simulink model "simulink_4"  (R2025b)
settings: Solver=ode45  StartTime=0.0  StopTime=0.5  MaxStep=1e-4  RelTol=1e-3
values from neighbouring files (symbols this model uses):
  A = [ -k1/(2*sqrt(x1e)),      0 ... (first row only)    [main.m]
  alpha = alpha_tau / tau    [main.m]
  B = [ k4; 0 ]    [main.m]
  C = [ 0, 1 ]    [main.m]
  D = 0    [main.m]
  Kr = 60    [main.m]
  tau = (M_star - cos(phi_rad)) / (wc_des * sin(phi_rad))    [main.m]
settings Model: Creator=porpo  LastModifiedBy=porpo

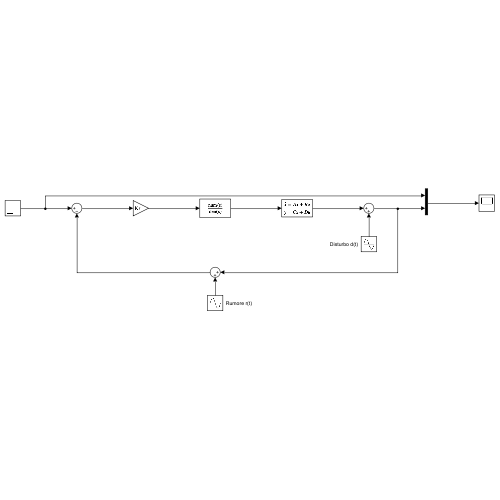
[thumbnail: Simulink's stored preview of the top-level diagram]
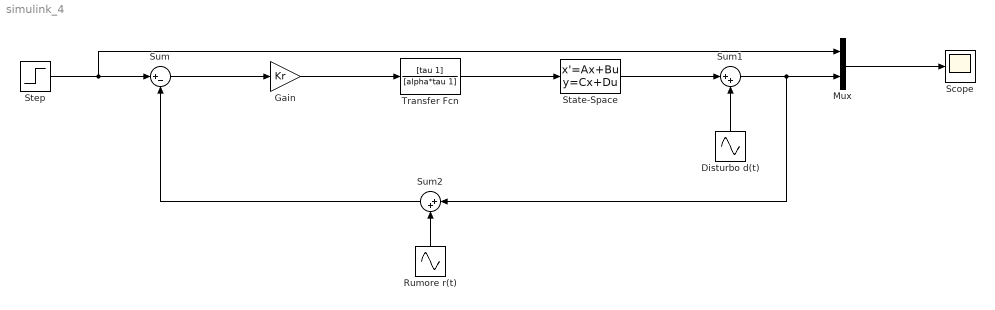
== system simulink_4 ==
  Disturbo d(t) : Sin  Amplitude=0  SampleTime=0
  Gain : Gain  Gain=Kr
  Mux : Mux  Inputs=2
  Rumore r(t) : Sin  Amplitude=0  SampleTime=0
  Scope : Scope
      settings: ActiveDisplayYMinimum=-0.95624767179996484  ActiveDisplayYMaximum=4.7591730752840817
  State-Space : StateSpace  A=A  B=B  C=C  D=D  InitialCondition=0
  Step : Step  Time=0  After=3  SampleTime=0
  Sum : Sum  Inputs=|+-
  Sum1 : Sum  Inputs=|++
  Sum2 : Sum  Inputs=|++
  Transfer Fcn : TransferFcn  Numerator=[tau 1]  Denominator=[alpha*tau 1]
  wires:
  Step/1 -> Mux/1, Sum/1
  Sum/1 -> Gain/1
  Gain/1 -> Transfer Fcn/1
  Transfer Fcn/1 -> State-Space/1
  State-Space/1 -> Sum1/1
  Disturbo d(t)/1 -> Sum1/2
  Sum1/1 -> Mux/2, Sum2/1
  Rumore r(t)/1 -> Sum2/2
  Sum2/1 -> Sum/2
  Mux/1 -> Scope/1
